simulink model "cart_ipd_sim"  (R2013a)
settings: Solver=ode4  SolverMode=SingleTasking  StartTime=0.0  StopTime=1  FixedStep=t_sim  RelTol=1e-3
values from neighbouring files (symbols this model uses):
  kD = (a2*wn - ac)/bc    [p2c242_ex2_cart_ipd.m]    (also in p2c242_ex2_cart_ipd_custom.m)
  kI = wn^3/bc    [p2c242_ex2_cart_ipd.m]    (also in p2c242_ex2_cart_ipd_custom.m)
  kP = a1*wn^2/bc    [p2c242_ex2_cart_ipd.m]    (also in p2c242_ex2_cart_ipd_custom.m)
  ts = 0.01    [p2c234_ex1_cdip_odq.m]    (also in p2c234_ex1_cdip_odq_custom.m; p2c242_ex2_cart_ipd.m = 0.025; p2c242_ex2_cart_ipd_custom.m = 0.025; p2c244_ex3_cdip_sampled_data_lqr_sim.m = 0.1)
undefined symbols (not defined in the file or in its folder): ac, bc
settings Model: Creator=kawata  LastModifiedBy=kawata
settings SolverCC: AutoInsertRateTranBlk=on  InsertRTBMode=Always
settings DataIOCC: SignalLoggingSaveFormat=ModelDataLogs
settings OptimizationCC: ExpressionDepthLimit=2147483647
settings DebuggingCC: FcnCallInpInsideContextMsg=UseLocalSettings
settings GRTTargetCC: CombineOutputUpdateFcns=off  GRTInterface=on

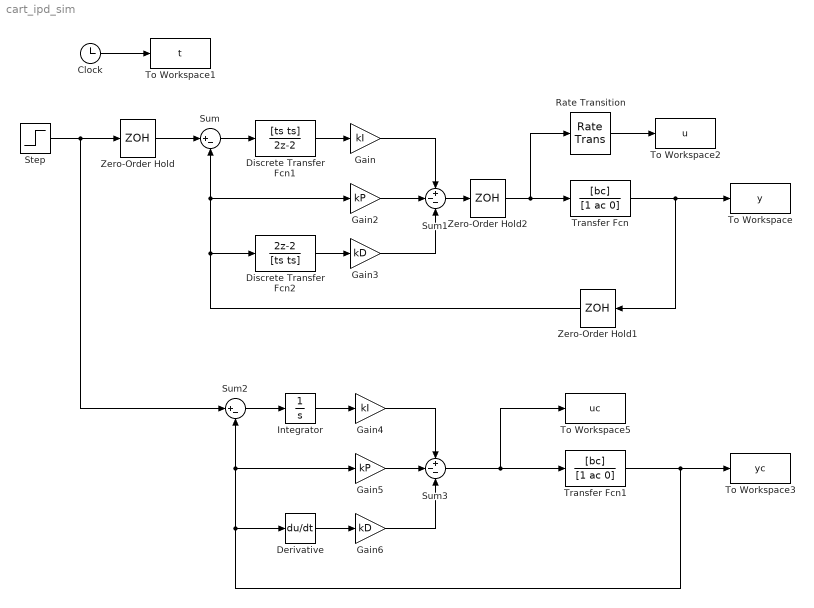
== system cart_ipd_sim ==
  Clock : Clock
  Derivative : Derivative
  Discrete Transfer Fcn1 : DiscreteTransferFcn  Numerator=[ts ts]  Denominator=[2 -2]  SampleTime=ts
  Discrete Transfer Fcn2 : DiscreteTransferFcn  Numerator=[2 -2]  Denominator=[ts ts]  SampleTime=ts
  Gain : Gain  Gain=kI
  Gain2 : Gain  Gain=kP
  Gain3 : Gain  Gain=kD
  Gain4 : Gain  Gain=kI
  Gain5 : Gain  Gain=kP
  Gain6 : Gain  Gain=kD
  Integrator : Integrator
  Rate Transition : RateTransition  OutPortSampleTime=t_sim
  Step : Step  Time=0  After=0.1  SampleTime=0
  Sum : Sum  Inputs=|+-
  Sum1 : Sum  Inputs=+--
  Sum2 : Sum  Inputs=|+-
  Sum3 : Sum  Inputs=+--
  To Workspace : ToWorkspace  VariableName=y  SampleTime=-1
  To Workspace1 : ToWorkspace  VariableName=t  SampleTime=-1
  To Workspace2 : ToWorkspace  VariableName=u  SampleTime=-1
  To Workspace3 : ToWorkspace  VariableName=yc  SampleTime=-1
  To Workspace5 : ToWorkspace  VariableName=uc  SampleTime=-1
  Transfer Fcn : TransferFcn  Numerator=[bc]  Denominator=[1 ac 0]
  Transfer Fcn1 : TransferFcn  Numerator=[bc]  Denominator=[1 ac 0]
  Zero-Order Hold : ZeroOrderHold  SampleTime=ts
  Zero-Order Hold1 : ZeroOrderHold  SampleTime=ts
  Zero-Order Hold2 : ZeroOrderHold  SampleTime=ts
  wires:
  Transfer Fcn/1 -> To Workspace/1, Zero-Order Hold1/1
  Discrete Transfer Fcn1/1 -> Gain/1
  Discrete Transfer Fcn2/1 -> Gain3/1
  Step/1 -> Sum2/1, Zero-Order Hold/1
  Clock/1 -> To Workspace1/1
  Sum3/1 -> To Workspace5/1, Transfer Fcn1/1
  Transfer Fcn1/1 -> To Workspace3/1, Sum2/2, Gain5/1, Derivative/1
  Integrator/1 -> Gain4/1
  Rate Transition/1 -> To Workspace2/1
  Sum2/1 -> Integrator/1
  Derivative/1 -> Gain6/1
  Gain4/1 -> Sum3/1
  Gain5/1 -> Sum3/2
  Gain6/1 -> Sum3/3
  Gain2/1 -> Sum1/2
  Gain3/1 -> Sum1/3
  Sum1/1 -> Zero-Order Hold2/1
  Gain/1 -> Sum1/1
  Sum/1 -> Discrete Transfer Fcn1/1
  Zero-Order Hold/1 -> Sum/1
  Zero-Order Hold1/1 -> Discrete Transfer Fcn2/1, Sum/2, Gain2/1
  Zero-Order Hold2/1 -> Transfer Fcn/1, Rate Transition/1
